simulink model "SerialMonitor"  (R2016a)
settings: Solver=ode3  StartTime=0.0  StopTime=100  FixedStep=.01  RelTol=1e-3
StartFcn:
  | s_2 = serial('COM10','BaudRate',115200,'FlowControl','none','Parity','none','DataBits',8,'StopBits',1,'Timeout',3);
  | s_2.InputBufferSize=1024; s_2.OutputBufferSize=1024;
  | s_2.Terminator='CR';
  | 
  | fopen(s_2);
StopFcn:
  | fclose(s_2);
undefined symbols (not defined in the file or in its folder): serialRead
settings Model: Creator=EliteBook 8470p  LastModifiedBy=rsjoshi1
settings DataIOCC: LimitDataPoints=on  SaveFormat=Array
settings DebuggingCC: SolverPrmCheckMsg=warning
settings HardwareCC: ProdBitPerPointer=32  ProdLargestAtomicFloat=None  ProdIntDivRoundTo=Undefined  ProdEndianess=Unspecified  ProdWordSize=32  ProdHWDeviceType=32-bit Generic
settings ModelReferenceCC: PropagateSignalLabelsOutOfModel=off
settings ConfigComp: CovModelRefEnable=Off  CovSFcnEnable=off

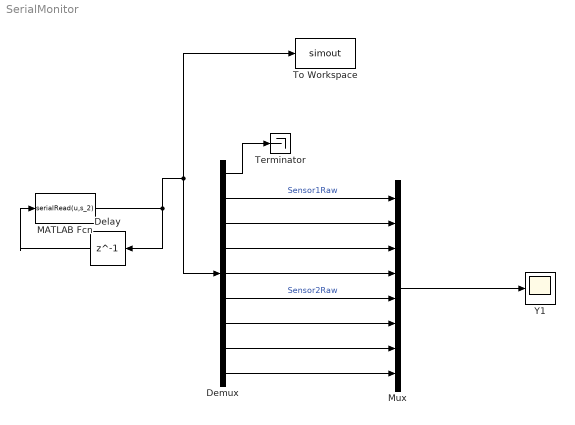
== system SerialMonitor ==
  Delay : Delay  DelayLength=1  InitialCondition=0
  Demux : Demux  Outputs=9
  MATLAB Fcn : MATLABFcn  MATLABFcn=serialRead(u,s_2)  OutputDimensions=9
  Mux : Mux  Inputs=8
  Terminator : Terminator
  To Workspace : ToWorkspace  VariableName=simout  SaveFormat=Timeseries  SampleTime=-1
  Y1 : Scope
  wires:
  Delay/1 -> MATLAB Fcn/1
  MATLAB Fcn/1 -> Delay/1, Demux/1, To Workspace/1
  Mux/1 -> Y1/1
  Demux/2 -> Mux/1  "Sensor1Raw"
  Demux/3 -> Mux/2
  Demux/4 -> Mux/3
  Demux/5 -> Mux/4
  Demux/6 -> Mux/5  "Sensor2Raw"
  Demux/7 -> Mux/6
  Demux/8 -> Mux/7
  Demux/9 -> Mux/8
  Demux/1 -> Terminator/1
